simulink model "Thermostat"  (R2024b)
settings: Solver=VariableStepAuto  StartTime=0.0  StopTime=1000  RelTol=1e-3
InitFcn:
  | % Room dimensions in meters
  | length = 2;  % length of the room (m)
  | width = 2;   % width of the room (m)
  | height = 3;  % height of the room (m)
  | 
  | % Air properties (approximate at 20°C)
  | rho = 1.2;   % air density (kg/m^3)
  | c_p = 1005;  % specific heat capacity of air (J/(kg*K))
  | 
  | % Heater scaling factor
  | k_u = 2000;  % heater power scaling (W)
  | 
  | % Thermal resistance
  | R = 1;      % thermal resistance (K/W)
  | 
  | % Temprature lost per timestep
  | lost_temp = 0.1;  % temperature lost per timestep (°C)
  | 
  | % Outside temperature (°C)
  | T_outside = 20;  % outside temperature (°C)
  | 
  | % Room volume (m^3)
  | V = length * width * height;  % volume of the room (m^3)
  | 
  | % Thermal capacitance (J/K)
  | C = rho * V * c_p;  % thermal capacitance (J/K)
settings Model: Creator=GAL98  LastModifiedBy=GAL98

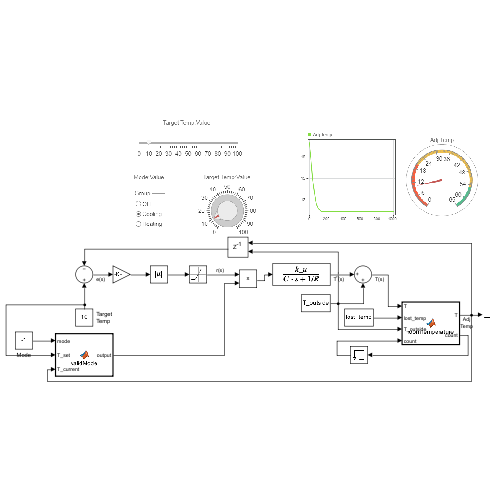
[thumbnail: Simulink's stored preview of the top-level diagram]
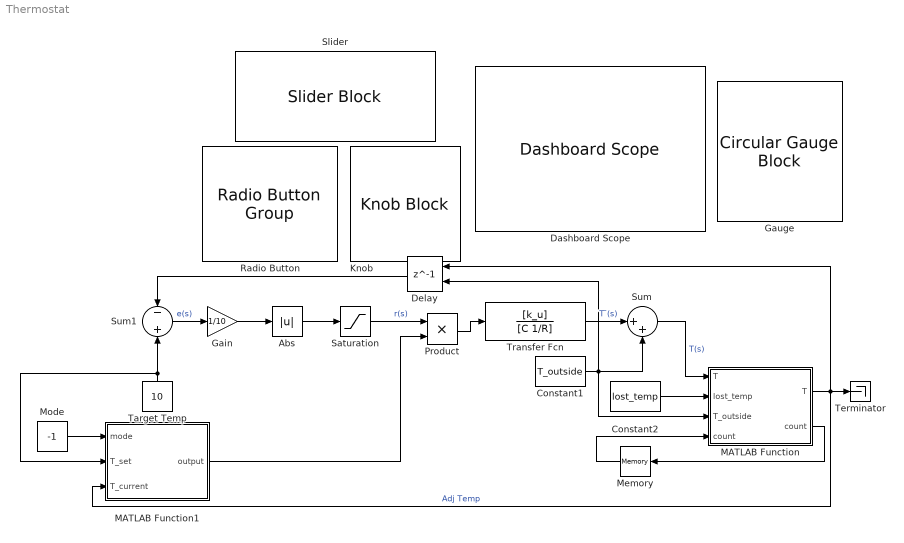
== system Thermostat ==
  Abs : Abs  SaturateOnIntegerOverflow=off
  Constant1 : Constant  Value=T_outside
  Constant2 : Constant  Value=lost_temp
  Dashboard Scope : DashboardScope  Ymin=0  Ymax=70  NormalizeYAxis=on
  Delay : Delay  DelayLength=1  InitialConditionSource=Input port  UseCircularBuffer=on
      settings: InputPortMap=u0,p4
  Gain : Gain  Gain=1/10
  Gauge : CircularGaugeBlock  ScaleMax=65
  Knob : KnobBlock
  MATLAB Function : MATLAB Function  TreatAsAtomicUnit=on
  MATLAB Function1 : MATLAB Function  TreatAsAtomicUnit=on
  Memory : Memory
  Mode : Constant  Value=-1
  Product : Product
  Radio Button : RadioButtonGroup  SelectedLabel=Cooling  ButtonGroupName=Group
      settings: Values={{'OFF', 'Cooling', 'Heating'}, [0 -1 1]}
  Saturation : Saturate  UpperLimit=1  LowerLimit=0
  Slider : SliderBlock
  Sum : Sum  Inputs=|++
  Sum1 : Sum  Inputs=-|+
  Target Temp : Constant  Value=10
  Terminator : Terminator
  Transfer Fcn : TransferFcn  Numerator=[k_u]  Denominator=[C 1/R]
  wires:
  Delay/1 -> Sum1/1
  MATLAB Function/2(count) -> Memory/1
  Target Temp/1 -> Sum1/2, MATLAB Function1/2(T_set)
  Memory/1 -> MATLAB Function/4("count ")
  Sum1/1 -> Gain/1  "e(s)"
  Saturation/1 -> Product/1  "r(s)"
  Transfer Fcn/1 -> Sum/1  "T ̃(s)"
  Constant1/1 -> Delay/2, MATLAB Function/3(T_outside), Sum/2
  Sum/1 -> MATLAB Function/1("T ")  "T(s)"
  Constant2/1 -> MATLAB Function/2(lost_temp)
  MATLAB Function/1(T) -> Delay/1, MATLAB Function1/3(T_current), Terminator/1  "Adj Temp"
  Gain/1 -> Abs/1
  Abs/1 -> Saturation/1
  Product/1 -> Transfer Fcn/1
  Mode/1 -> MATLAB Function1/1(mode)
  MATLAB Function1/1(output) -> Product/2

== matlab function Thermostat/MATLAB Function1 ==
  data: mode input; T_set input; T_current input; output output
function output  = validMode(mode, T_set, T_current)
    % validMode: Ensures heating or cooling mode is valid based on temperature conditions
    %
    % Inputs:
    %   mode - Desired operation mode (1 for heating, -1 for cooling)
    %   T_set - Setpoint temperature (°C)
    %   T_current - Current room temperature (°C)
    %
    % Output:
    %   output - Adjusted mode (1 for heating, -1 for cooling, 0 if invalid)
    
    % Check for invalid conditions
    if (mode == 1 && T_set < T_current) || (mode == -1 && T_set > T_current)
        output = 0;  % Invalid operation, no heating/cooling needed
    else
        output = mode;  % Valid operation, proceed with heating or cooling
    end
end

== matlab function Thermostat/MATLAB Function ==
  data: T input; lost_temp input; T_outside input; T output; count input; count output
function [T, count] = roomTemperature(T, lost_temp, T_outside, count)
    % roomTemperature: Adjusts the room temperature based on temperature reduction criteria
    %
    % Inputs:
    %   T - Current room temperature (°C)
    %   lost_temp - Temperature change per timestep (°C)
    %   T_outside - Outside temperature (°C)
    %   count - Counter tracking time spent adjusting the temperature
    %
    % Outputs:
    %   T - Adjusted room temperature (°C)
    %   count - Updated counter for time spent in temperature adjustment
    
    % Case 1: Room temperature is greater than outside temperature
    if T > T_outside
        % Check if the temperature can still be reduced
        if T - (lost_temp * count) > T_outside
            T = T - (lost_temp * count);  % Reduce temperature based on the count
            count = count + 1;  % Increment the counter for each timestep above outside temperature
        else
            % If the room temperature reaches or falls below outside temperature, stop reducing
            count = 0;  % Reset the counter as no further reduction is needed
            T = T_outside;  % Set temperature to outside temperature
        end
        
    % Case 2: Room temperature is less than outside temperature
    elseif T < T_outside
        % Check if the temperature can still increase towards the outside temperature
        if T + (lost_temp * count) < T_outside
            T = T + (lost_temp * count);  % Increase temperature based on the count
            count = count + 1;  % Increment the counter for each timestep the temperature is below outside
        else
            % If the room temperature reaches or exceeds outside temperature, stop increasing
            count = 0;  % Reset the counter as no further increase is needed
            T = T_outside;  % Set temperature to outside temperature
        end
        
    % Case 3: Room temperature is equal to outside temperature
    else
        count = 0;  % No temperature adjustment is needed when T equals T_outside
    end
end
